simulink model "modelo_sistema"  (R2018b)
settings: Solver=ode3  StartTime=0.0  StopTime=10.0  FixedStep=1e-3  RelTol=1e-3
values from neighbouring files (symbols this model uses):
  A = 6.597e-3    (= 0.006597)    [params_2.m]
  amp = amps(a)    [params_2.m]
  Kq0 = 2.15    [params_2.m]
  l1 = 0.1    [params_2.m]
  l2 = razoes(r)*l1    [params_2.m]
settings Model: Creator=yasminnunes  LastModifiedBy=yasminnunes

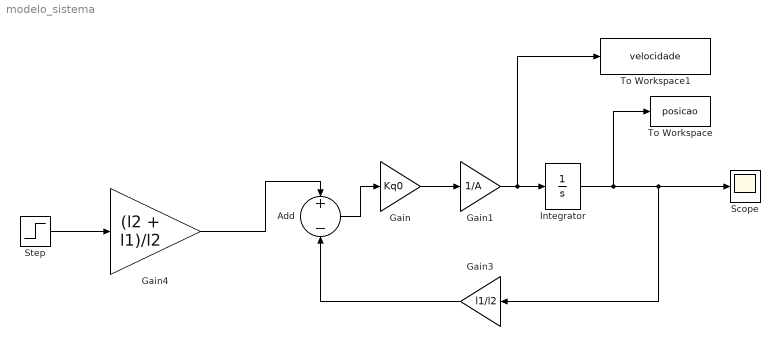
== system modelo_sistema ==
  Add : Sum  Inputs=+-
  Gain : Gain  Gain=Kq0
  Gain1 : Gain  Gain=1/A
  Gain3 : Gain  Gain=l1/l2
  Gain4 : Gain  Gain=(l2 + l1)/l2
  Integrator : Integrator
  Scope : Scope
  Step : Step  After=amp  SampleTime=0
  To Workspace : ToWorkspace  VariableName=posicao  SaveFormat=Timeseries  SampleTime=-1
  To Workspace1 : ToWorkspace  VariableName=velocidade  SaveFormat=Timeseries  SampleTime=-1
  wires:
  Add/1 -> Gain/1
  Gain/1 -> Gain1/1
  Gain1/1 -> To Workspace1/1, Integrator/1
  Integrator/1 -> To Workspace/1, Scope/1, Gain3/1
  Gain3/1 -> Add/2
  Gain4/1 -> Add/1
  Step/1 -> Gain4/1
